simulink model "Real_ECU"  (R2016b)
settings: Solver=FixedStepDiscrete  StartTime=0.0  StopTime=inf  FixedStep=RealECU.tiSimnTiStep_C  RelTol=1e-3  EnableMultiTasking=on
settings Model: Creator=m01wolf  LastModifiedBy=bunver
settings DataIOCC: SaveFormat=StructureWithTime  SaveOutput=off  DSMLogging=off  VisualizeSimOutput=off  SaveTime=off  SignalLoggingName=Results
settings OptimizationCC: BlockReduction=off  ConditionallyExecuteInputs=off  LifeSpan=inf
settings DebuggingCC: AllowSymbolicDim=off  SFUnexpectedBacktrackingDiag=warning  SFNoUnconditionalDefaultTransitionDiag=warning  SFExecutionAtInitializationDiag=none
settings ModelReferenceCC: ModelReferenceNumInstancesAllowed=Single  PropagateSignalLabelsOutOfModel=off
settings GRTTargetCC: TargetLangStandard=C89/C90 (ANSI)
settings ConfigComp: CovMetricSettings=dw  CovHtmlReporting=on  CovSaveCumulativeToWorkspaceVar=on  CovSaveSingleToWorkspaceVar=on  CovExternalEMLEnable=off

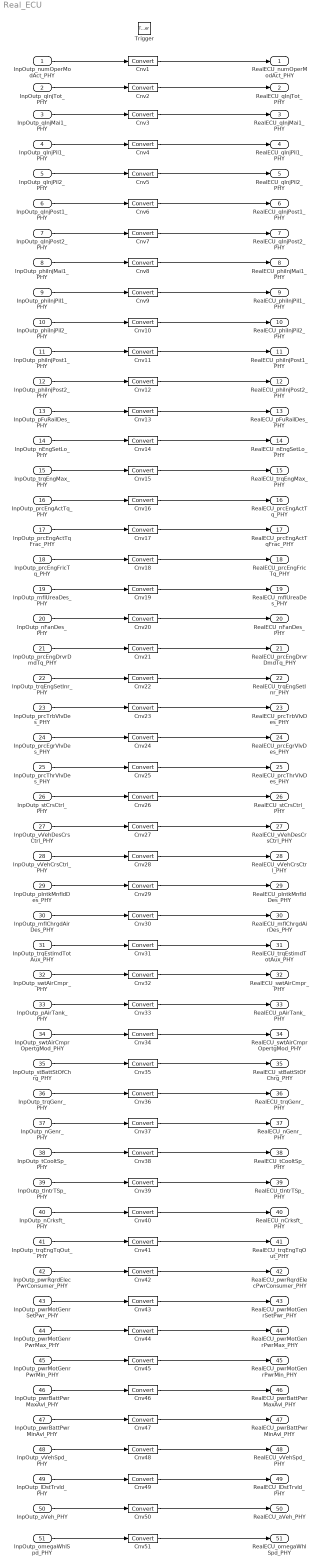
== system Real_ECU ==
  InpOutp_numOperModAct_PHY : Inport
  InpOutp_qInjTot_PHY : Inport  Port=2
  InpOutp_qInjMai1_PHY : Inport  Port=3
  InpOutp_qInjPil1_PHY : Inport  Port=4
  InpOutp_qInjPil2_PHY : Inport  Port=5
  InpOutp_qInjPost1_PHY : Inport  Port=6
  InpOutp_qInjPost2_PHY : Inport  Port=7
  InpOutp_phiInjMai1_PHY : Inport  Port=8
  InpOutp_phiInjPil1_PHY : Inport  Port=9
  InpOutp_phiInjPil2_PHY : Inport  Port=10
  InpOutp_phiInjPost1_PHY : Inport  Port=11
  InpOutp_phiInjPost2_PHY : Inport  Port=12
  InpOutp_pFuRailDes_PHY : Inport  Port=13
  InpOutp_nEngSetLo_PHY : Inport  Port=14
  InpOutp_trqEngMax_PHY : Inport  Port=15
  InpOutp_prcEngActTq_PHY : Inport  Port=16
  InpOutp_prcEngActTqFrac_PHY : Inport  Port=17
  InpOutp_prcEngFricTq_PHY : Inport  Port=18
  InpOutp_mflUreaDes_PHY : Inport  Port=19
  InpOutp_nFanDes_PHY : Inport  Port=20
  InpOutp_prcEngDrvrDmdTq_PHY : Inport  Port=21
  InpOutp_trqEngSetInr_PHY : Inport  Port=22
  InpOutp_prcTrbVlvDes_PHY : Inport  Port=23
  InpOutp_prcEgrVlvDes_PHY : Inport  Port=24
  InpOutp_prcThrVlvDes_PHY : Inport  Port=25
  InpOutp_stCrsCtrl_PHY : Inport  Port=26
  InpOutp_vVehDesCrsCtrl_PHY : Inport  Port=27
  InpOutp_vVehCrsCtrl_PHY : Inport  Port=28
  InpOutp_pIntkMnfldDes_PHY : Inport  Port=29
  InpOutp_mflChrgdAirDes_PHY : Inport  Port=30
  InpOutp_trqEstimdTotAux_PHY : Inport  Port=31
  InpOutp_swtAirCmpr_PHY : Inport  Port=32
  InpOutp_pAirTank_PHY : Inport  Port=33
  InpOutp_swtAirCmprOpertgMod_PHY : Inport  Port=34
  InpOutp_stBattStOfChrg_PHY : Inport  Port=35
  InpOutp_trqGenr_PHY : Inport  Port=36
  InpOutp_nGenr_PHY : Inport  Port=37
  InpOutp_tCooltSp_PHY : Inport  Port=38
  InpOutp_tIntrTSp_PHY : Inport  Port=39
  InpOutp_nCrksft_PHY : Inport  Port=40
  InpOutp_trqEngTqOut_PHY : Inport  Port=41
  InpOutp_pwrRqrdElecPwrConsumer_PHY : Inport  Port=42
  InpOutp_pwrMotGenrSetPwr_PHY : Inport  Port=43
  InpOutp_pwrMotGenrPwrMax_PHY : Inport  Port=44
  InpOutp_pwrMotGenrPwrMin_PHY : Inport  Port=45
  InpOutp_pwrBattPwrMaxAvl_PHY : Inport  Port=46
  InpOutp_pwrBattPwrMinAvl_PHY : Inport  Port=47
  InpOutp_vVehSpd_PHY : Inport  Port=48
  InpOutp_lDstTrvld_PHY : Inport  Port=49
  InpOutp_aVeh_PHY : Inport  Port=50
  InpOutp_omegaWhlSpd_PHY : Inport  Port=51
  Trigger : TriggerPort  TriggerType=function-call  VariantControl=Variant  PortDimensions=1
  Cnv{1..51} (51 alike) : DataTypeConversion
  RealECU_numOperModAct_PHY : Outport
  RealECU_qInjTot_PHY : Outport  Port=2
  RealECU_qInjMai1_PHY : Outport  Port=3
  RealECU_qInjPil1_PHY : Outport  Port=4
  RealECU_qInjPil2_PHY : Outport  Port=5
  RealECU_qInjPost1_PHY : Outport  Port=6
  RealECU_qInjPost2_PHY : Outport  Port=7
  RealECU_phiInjMai1_PHY : Outport  Port=8
  RealECU_phiInjPil1_PHY : Outport  Port=9
  RealECU_phiInjPil2_PHY : Outport  Port=10
  RealECU_phiInjPost1_PHY : Outport  Port=11
  RealECU_phiInjPost2_PHY : Outport  Port=12
  RealECU_pFuRailDes_PHY : Outport  Port=13
  RealECU_nEngSetLo_PHY : Outport  Port=14
  RealECU_trqEngMax_PHY : Outport  Port=15
  RealECU_prcEngActTq_PHY : Outport  Port=16
  RealECU_prcEngActTqFrac_PHY : Outport  Port=17
  RealECU_prcEngFricTq_PHY : Outport  Port=18
  RealECU_mflUreaDes_PHY : Outport  Port=19
  RealECU_nFanDes_PHY : Outport  Port=20
  RealECU_prcEngDrvrDmdTq_PHY : Outport  Port=21
  RealECU_trqEngSetInr_PHY : Outport  Port=22
  RealECU_prcTrbVlvDes_PHY : Outport  Port=23
  RealECU_prcEgrVlvDes_PHY : Outport  Port=24
  RealECU_prcThrVlvDes_PHY : Outport  Port=25
  RealECU_stCrsCtrl_PHY : Outport  Port=26
  RealECU_vVehDesCrsCtrl_PHY : Outport  Port=27
  RealECU_vVehCrsCtrl_PHY : Outport  Port=28
  RealECU_pIntkMnfldDes_PHY : Outport  Port=29
  RealECU_mflChrgdAirDes_PHY : Outport  Port=30
  RealECU_trqEstimdTotAux_PHY : Outport  Port=31
  RealECU_swtAirCmpr_PHY : Outport  Port=32
  RealECU_pAirTank_PHY : Outport  Port=33
  RealECU_swtAirCmprOpertgMod_PHY : Outport  Port=34
  RealECU_stBattStOfChrg_PHY : Outport  Port=35
  RealECU_trqGenr_PHY : Outport  Port=36
  RealECU_nGenr_PHY : Outport  Port=37
  RealECU_tCooltSp_PHY : Outport  Port=38
  RealECU_tIntrTSp_PHY : Outport  Port=39
  RealECU_nCrksft_PHY : Outport  Port=40
  RealECU_trqEngTqOut_PHY : Outport  Port=41
  RealECU_pwrRqrdElecPwrConsumer_PHY : Outport  Port=42
  RealECU_pwrMotGenrSetPwr_PHY : Outport  Port=43
  RealECU_pwrMotGenrPwrMax_PHY : Outport  Port=44
  RealECU_pwrMotGenrPwrMin_PHY : Outport  Port=45
  RealECU_pwrBattPwrMaxAvl_PHY : Outport  Port=46
  RealECU_pwrBattPwrMinAvl_PHY : Outport  Port=47
  RealECU_vVehSpd_PHY : Outport  Port=48
  RealECU_lDstTrvld_PHY : Outport  Port=49
  RealECU_aVeh_PHY : Outport  Port=50
  RealECU_omegaWhlSpd_PHY : Outport  Port=51
  wires:
  InpOutp_numOperModAct_PHY/1 -> Cnv1/1
  InpOutp_qInjTot_PHY/1 -> Cnv2/1
  InpOutp_qInjMai1_PHY/1 -> Cnv3/1
  InpOutp_qInjPil1_PHY/1 -> Cnv4/1
  InpOutp_qInjPil2_PHY/1 -> Cnv5/1
  InpOutp_qInjPost1_PHY/1 -> Cnv6/1
  InpOutp_qInjPost2_PHY/1 -> Cnv7/1
  InpOutp_phiInjMai1_PHY/1 -> Cnv8/1
  InpOutp_phiInjPil1_PHY/1 -> Cnv9/1
  InpOutp_phiInjPil2_PHY/1 -> Cnv10/1
  InpOutp_phiInjPost1_PHY/1 -> Cnv11/1
  InpOutp_phiInjPost2_PHY/1 -> Cnv12/1
  InpOutp_pFuRailDes_PHY/1 -> Cnv13/1
  InpOutp_nEngSetLo_PHY/1 -> Cnv14/1
  InpOutp_trqEngMax_PHY/1 -> Cnv15/1
  InpOutp_prcEngActTq_PHY/1 -> Cnv16/1
  InpOutp_prcEngActTqFrac_PHY/1 -> Cnv17/1
  InpOutp_prcEngFricTq_PHY/1 -> Cnv18/1
  InpOutp_mflUreaDes_PHY/1 -> Cnv19/1
  InpOutp_nFanDes_PHY/1 -> Cnv20/1
  InpOutp_prcEngDrvrDmdTq_PHY/1 -> Cnv21/1
  InpOutp_trqEngSetInr_PHY/1 -> Cnv22/1
  InpOutp_prcTrbVlvDes_PHY/1 -> Cnv23/1
  InpOutp_prcEgrVlvDes_PHY/1 -> Cnv24/1
  InpOutp_prcThrVlvDes_PHY/1 -> Cnv25/1
  InpOutp_stCrsCtrl_PHY/1 -> Cnv26/1
  InpOutp_vVehDesCrsCtrl_PHY/1 -> Cnv27/1
  InpOutp_vVehCrsCtrl_PHY/1 -> Cnv28/1
  InpOutp_pIntkMnfldDes_PHY/1 -> Cnv29/1
  InpOutp_mflChrgdAirDes_PHY/1 -> Cnv30/1
  InpOutp_trqEstimdTotAux_PHY/1 -> Cnv31/1
  InpOutp_swtAirCmpr_PHY/1 -> Cnv32/1
  InpOutp_pAirTank_PHY/1 -> Cnv33/1
  InpOutp_swtAirCmprOpertgMod_PHY/1 -> Cnv34/1
  InpOutp_stBattStOfChrg_PHY/1 -> Cnv35/1
  InpOutp_trqGenr_PHY/1 -> Cnv36/1
  InpOutp_nGenr_PHY/1 -> Cnv37/1
  InpOutp_tCooltSp_PHY/1 -> Cnv38/1
  InpOutp_tIntrTSp_PHY/1 -> Cnv39/1
  InpOutp_nCrksft_PHY/1 -> Cnv40/1
  InpOutp_trqEngTqOut_PHY/1 -> Cnv41/1
  InpOutp_pwrRqrdElecPwrConsumer_PHY/1 -> Cnv42/1
  InpOutp_pwrMotGenrSetPwr_PHY/1 -> Cnv43/1
  InpOutp_pwrMotGenrPwrMax_PHY/1 -> Cnv44/1
  InpOutp_pwrMotGenrPwrMin_PHY/1 -> Cnv45/1
  InpOutp_pwrBattPwrMaxAvl_PHY/1 -> Cnv46/1
  InpOutp_pwrBattPwrMinAvl_PHY/1 -> Cnv47/1
  InpOutp_vVehSpd_PHY/1 -> Cnv48/1
  InpOutp_lDstTrvld_PHY/1 -> Cnv49/1
  InpOutp_aVeh_PHY/1 -> Cnv50/1
  InpOutp_omegaWhlSpd_PHY/1 -> Cnv51/1
  Cnv1/1 -> RealECU_numOperModAct_PHY/1
  Cnv2/1 -> RealECU_qInjTot_PHY/1
  Cnv3/1 -> RealECU_qInjMai1_PHY/1
  Cnv4/1 -> RealECU_qInjPil1_PHY/1
  Cnv5/1 -> RealECU_qInjPil2_PHY/1
  Cnv6/1 -> RealECU_qInjPost1_PHY/1
  Cnv51/1 -> RealECU_omegaWhlSpd_PHY/1
  Cnv7/1 -> RealECU_qInjPost2_PHY/1
  Cnv8/1 -> RealECU_phiInjMai1_PHY/1
  Cnv9/1 -> RealECU_phiInjPil1_PHY/1
  Cnv10/1 -> RealECU_phiInjPil2_PHY/1
  Cnv11/1 -> RealECU_phiInjPost1_PHY/1
  Cnv12/1 -> RealECU_phiInjPost2_PHY/1
  Cnv13/1 -> RealECU_pFuRailDes_PHY/1
  Cnv14/1 -> RealECU_nEngSetLo_PHY/1
  Cnv15/1 -> RealECU_trqEngMax_PHY/1
  Cnv16/1 -> RealECU_prcEngActTq_PHY/1
  Cnv17/1 -> RealECU_prcEngActTqFrac_PHY/1
  Cnv18/1 -> RealECU_prcEngFricTq_PHY/1
  Cnv19/1 -> RealECU_mflUreaDes_PHY/1
  Cnv20/1 -> RealECU_nFanDes_PHY/1
  Cnv21/1 -> RealECU_prcEngDrvrDmdTq_PHY/1
  Cnv22/1 -> RealECU_trqEngSetInr_PHY/1
  Cnv23/1 -> RealECU_prcTrbVlvDes_PHY/1
  Cnv24/1 -> RealECU_prcEgrVlvDes_PHY/1
  Cnv25/1 -> RealECU_prcThrVlvDes_PHY/1
  Cnv26/1 -> RealECU_stCrsCtrl_PHY/1
  Cnv27/1 -> RealECU_vVehDesCrsCtrl_PHY/1
  Cnv28/1 -> RealECU_vVehCrsCtrl_PHY/1
  Cnv29/1 -> RealECU_pIntkMnfldDes_PHY/1
  Cnv30/1 -> RealECU_mflChrgdAirDes_PHY/1
  Cnv31/1 -> RealECU_trqEstimdTotAux_PHY/1
  Cnv32/1 -> RealECU_swtAirCmpr_PHY/1
  Cnv33/1 -> RealECU_pAirTank_PHY/1
  Cnv34/1 -> RealECU_swtAirCmprOpertgMod_PHY/1
  Cnv35/1 -> RealECU_stBattStOfChrg_PHY/1
  Cnv36/1 -> RealECU_trqGenr_PHY/1
  Cnv37/1 -> RealECU_nGenr_PHY/1
  Cnv38/1 -> RealECU_tCooltSp_PHY/1
  Cnv39/1 -> RealECU_tIntrTSp_PHY/1
  Cnv40/1 -> RealECU_nCrksft_PHY/1
  Cnv42/1 -> RealECU_pwrRqrdElecPwrConsumer_PHY/1
  Cnv41/1 -> RealECU_trqEngTqOut_PHY/1
  Cnv43/1 -> RealECU_pwrMotGenrSetPwr_PHY/1
  Cnv44/1 -> RealECU_pwrMotGenrPwrMax_PHY/1
  Cnv45/1 -> RealECU_pwrMotGenrPwrMin_PHY/1
  Cnv46/1 -> RealECU_pwrBattPwrMaxAvl_PHY/1
  Cnv47/1 -> RealECU_pwrBattPwrMinAvl_PHY/1
  Cnv48/1 -> RealECU_vVehSpd_PHY/1
  Cnv49/1 -> RealECU_lDstTrvld_PHY/1
  Cnv50/1 -> RealECU_aVeh_PHY/1
